simulink model "SSVEPrealtime2017"  (R2017a)
settings: Solver=VariableStepAuto  StartTime=0.0  StopTime=inf  RelTol=1e-3
libraries: dspindex x2, dspnetwork x1
settings Model: Creator=Jskyl  LastModifiedBy=a436q344
settings SFSimCC: SimUseLocalCustomCode=on
settings RTWCC: RTWUseLocalCustomCode=on

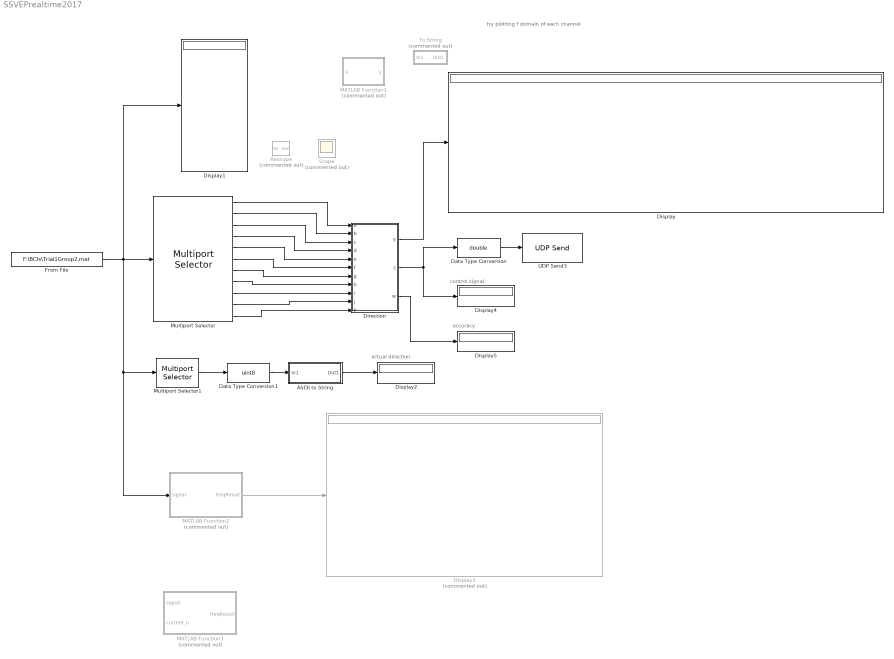
== system SSVEPrealtime2017 ==
  note: try plotting f domain of each channel
  note: actual direction
  note: accuracy
  note: control signal
  ASCII to String : Subsystem  Description=Replaced Block  mask(Replaced Block){}
      mask help: This block has been replaced with an empty subsystem because it used functionality that is unavailable in Simulink R2017a.
      mask Display: fprintf('Replaced: %s\n','ASCIIToString')
  Data Type Conversion : DataTypeConversion  OutDataTypeStr=double  ConvertRealWorld=Stored Integer (SI)
  Data Type Conversion1 : DataTypeConversion  OutDataTypeStr=uint8
  Direction : MATLAB Function  TreatAsAtomicUnit=on
  Display{,1..2,4..5} (5 alike) : Display
  Display3 : Display  Commented=on
  From File : FromFile  FileName=F:\BCIs\Trial1Group2.mat  OutDataTypeStr=double  SampleTime=1/512
  MATLAB Function1 : MATLAB Function  Commented=on  TreatAsAtomicUnit=on
  MATLAB Function2 : MATLAB Function  Commented=on  TreatAsAtomicUnit=on
  MATLAB Function3 : MATLAB Function  Commented=on  TreatAsAtomicUnit=on
  Multiport Selector : dspindex/Multiport Selector  rowsOrCols=Rows  idxCellArray={ 1,2,3,4,5,6,7,8,9,10,11 }  idxErrMode=Clip Index
  Multiport Selector1 : dspindex/Multiport Selector  rowsOrCols=Rows  idxCellArray={ 11 }  idxErrMode=Clip Index
  Reshape : Reshape  Commented=on  OutputDimensionality=Customize  OutputDimensions=[10,1]
  Scope : Scope  Commented=on
  To String : Subsystem  Description=Replaced Block  Commented=on  mask(Replaced Block){}
      mask help: This block has been replaced with an empty subsystem because it used functionality that is unavailable in Simulink R2017a.
      mask Display: fprintf('Replaced: %s\n','ToString')
  UDP Send3 : dspnetwork/UDP Send  remoteURL='127.0.0.1'  remotePort=25000  localURL='0.0.0.0'  localPortSource=Automatically determine  localPort=-1  sampletime=-1  blockPlatform=[]  separateLengthPort=0
  wires:
  Direction/1(y) -> Display/1
  From File/1 -> MATLAB Function2/1(signal), Multiport Selector1/1, Display1/1, Multiport Selector/1
  ASCII to String/1(Out1) -> Display2/1
  Multiport Selector1/1 -> Data Type Conversion1/1
  Data Type Conversion1/1 -> ASCII to String/1(In1)
  Multiport Selector/1 -> Direction/1(a)
  Multiport Selector/2 -> Direction/2(b)
  Multiport Selector/3 -> Direction/3(c)
  Multiport Selector/4 -> Direction/4(d)
  Multiport Selector/5 -> Direction/5(e)
  Multiport Selector/6 -> Direction/6(f)
  Multiport Selector/7 -> Direction/7(g)
  Multiport Selector/8 -> Direction/8(h)
  Multiport Selector/9 -> Direction/9(i)
  Multiport Selector/10 -> Direction/10(j)
  MATLAB Function2/1(freqResult) -> Display3/1
  Multiport Selector/11 -> Direction/11(k)
  Data Type Conversion/1 -> UDP Send3/1
  Direction/2(z) -> Display4/1, Data Type Conversion/1
  Direction/3(w) -> Display5/1

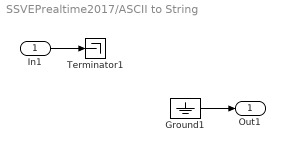
== system SSVEPrealtime2017/ASCII to String ==
  In1 : Inport
  Ground1 : Ground
  Terminator1 : Terminator
  Out1 : Outport
  wires:
  Ground1/1 -> Out1/1
  In1/1 -> Terminator1/1

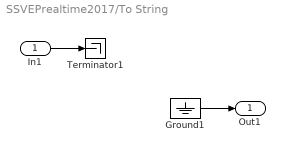
== system SSVEPrealtime2017/To String ==
  In1 : Inport
  Ground1 : Ground
  Terminator1 : Terminator
  Out1 : Outport
  wires:
  Ground1/1 -> Out1/1
  In1/1 -> Terminator1/1

== matlab function SSVEPrealtime2017/Direction ==
  data: y output size=[10 513]; a input; b input; c input; d input; e input; f input; g input; h input; i input; j input; k input; z output; w output
function [y,z,w]= fcn(a,b,c,d,e,f,g,h,i,j,k)

u = [a;b;c;d;e;f;g;h;i;j];
freq = [11 13.5 16 18.5 21 23.5 25];

persistent v
if isempty(v)
    v = 100;
end

persistent x
if isempty(x)
    x = 102;
end

persistent dir
if isempty(dir)
    dir = k;
end

persistent acc
if isempty(acc)
    acc = 0;
end

persistent keep
if isempty(keep)
   keep = 0; 
end

persistent n
if isempty(n)
    n = 0;
end

persistent mat
if isempty(mat)
    mat = u;
end

n = n + 1;
mat = [mat u]; %(1:10,n)

if k ~= 102
    dir = [dir k];
end

y = mat;

constant = 1;
sampleRate = 512;
f = constant*(0:(sampleRate/2));

%xMaxC1 = zeros(512);

if length(mat) == 513
    lowEnd = 9;
    highEnd = 31;
    filterOrder = 4; %how does this affect the outcome?
    [b,a] = butter(filterOrder, [lowEnd highEnd]/(sampleRate/2));
    data1 = filtfilt(b, a, y(1,:));
    data2 = filtfilt(b, a, y(2,:));
    data3 = filtfilt(b, a, y(3,:));
    data4 = filtfilt(b, a, y(4,:));
    data5 = filtfilt(b, a, y(5,:));
    data6 = filtfilt(b, a, y(6,:));
    data7 = filtfilt(b, a, y(7,:));
    data8 = filtfilt(b, a, y(8,:));
    data9 = filtfilt(b, a, y(9,:));
    data10 = filtfilt(b, a, y(10,:));

    y = [data1; data2; data3; data4; data5; data6; data7; data8; data9; data10];
    
    fftC1 = fft(y(1,:), 512); % C1
    pfftC1 = abs(fftC1);
    [maxC1, iMaxC1] = max(pfftC1);
    xMaxC1 = f(iMaxC1);
    fftC2 = abs(fft(y(2,:), 512)); % C2
    [maxC2, iMaxC2] = max(fftC2);
    xMaxC2 = f(iMaxC2);
    fftC3 = abs(fft(y(3,:), 512)); % C3
    [maxC3, iMaxC3] = max(fftC3);
    xMaxC3 = f(iMaxC3);
    fftC4 = abs(fft(y(4,:), 512)); % C4
    [maxC4, iMaxC4] = max(fftC4);
    xMaxC4= f(iMaxC4);
    fftC5 = abs(fft(y(5,:), 512)); % C5
    [maxC5, iMaxC5] = max(fftC5);
    xMaxC5 = f(iMaxC5);
    fftC6 = abs(fft(y(6,:), 512)); % C6
    [maxC6, iMaxC6] = max(fftC6);
    xMaxC6 = f(iMaxC6);
    fftC7 = abs(fft(y(7,:), 512)); % C7
    [maxC7, iMaxC7] = max(fftC7);
    xMaxC7 = f(iMaxC7);
    fftC8 = abs(fft(y(8,:), 512)); % C8
    [maxC8, iMaxC8] = max(fftC8);
    xMaxC8 = f(iMaxC8);
    fftC9 = abs(fft(y(9,:), 512)); % C9
    [maxC9, iMaxC9] = max(fftC9);
    xMaxC9 = f(iMaxC9);
    fftC10 = abs(fft(y(10,:), 512)); % C10
    [maxC10, iMaxC10] = max(fftC10);
    xMaxC10 = f(iMaxC10);

    xMax = [xMaxC1 xMaxC2 xMaxC3 xMaxC4 xMaxC5 xMaxC6 xMaxC7 xMaxC8 xMaxC9 xMaxC10];
    xMaxAvg = mean(xMax);
    keep = [keep xMaxAvg]
    
    %average
    
    direction = abs(xMaxAvg - freq);
    [minDirection, iDirection] = min(direction);
    
    if iDirection == 1
        z = 117;
        x = z;
        disp('up');
        if mode(dir) == 117
            acc = [acc 1];
        else
            acc = [acc 0];
        end
    end
    if iDirection == 2
        z = 105;
        x = z;
        disp('in');
        if mode(dir) == 105
            acc = [acc 1];
        else
            acc = [acc 0];
        end
    end
    if iDirection == 3
        z = 114;
        x = z;
        disp('right');
        if mode(dir) == 114
            acc = [acc 1];
        else
            acc = [acc 0];
        end
    end
    if iDirection == 4
        z = 100;
        x = z;
        disp('down');
        if mode(dir) == 100
            acc = [acc 1];
        else
            acc = [acc 0];
        end
    end
    if iDirection == 5
        z = 111;
        x = z;
        disp('out');
        if mode(dir) == 111
            acc = [acc 1];
        else
            acc = [acc 0];
        end
    end
    if iDirection == 6
        z = 108;
        x = z;
        disp('left');
        if mode(dir) == 108
            acc = [acc 1];
        else
            acc = [acc 0];
        end
    end
    if iDirection == 7
        z = 115;
        x = z;
        disp('stop');
        if mode(dir) == 115
            acc = [acc 1];
        else
            acc = [acc 0];
        end
    end
    
    %dispDir = sprintf('Direction = %f' , mode(dir));
    %disp(dispDir);
    disp(mode(dir));
    
    accuracy = 100*sum(acc)/(length(acc)-1);
    %dispAcc = sprintf('Accuracy = %.3f' , accuracy);
    %disp(accuracy);
    v = accuracy;
end

w = v;
z = x;

if n == 512
    mat = u;
    n = 0;
    dir = k;
    %acc = 0;
    %disp("done");
end

== matlab function SSVEPrealtime2017/MATLAB Function1 ==
  data: u input; y output
function y = fcn(u)

string var;

if u == 108
   var = "left";
end
if u == 102
   var = "right";
end
if u == 117
   var = "up";
end
if u == 100
   var = "down";
end
if u == 105
   var = "in";
end
if u == 111
   var = "out";
end
if u == 115
   var = "stop";
end
if u == 102
   var = "off";
end

y = double(charg(var));

== matlab function SSVEPrealtime2017/MATLAB Function2 ==
  data: signal input; freqResult output
function freqResult=MEC(signal) %current_n

signal=signal';
%% Functions Enabling 
CMA_filter=1;
FFT_HP_IFFT=1;
exp_transform=0;
mid_freqs=1;
consider_threshhold=0;

%% Defining Parameteres

f=[11 13.5 16 18.5 21 23.5 25];            %frequencies in concern
Fs = 128;           %Sampling frequency of Emotive
O1=7;               %| Name and number of channals 
O2=8;
T7=5;
T8=10;
Nh=2;               %#of Harmonics 
Ny=4;               %#of using Channals
alfa_energy_co=0.25;    %alfa as in the last section of paper#3
beta_classification=0.35;    %beta as in the last section of paper#3
valid_channal=[1 2 3 4 6 9 11 12 13 14]; %Valid Channals except using channals (O1, O2, T7 , T8) to use in CMA
cutting_freq=5;  %freq at which HP filter work

%% Calculating Needed Parameteres 
if (mid_freqs)
    %freqs in concern (including mid Freqs)
    midFreq=diff(f)/2+f(1:length(f)-1);
    f=horzcat(f,midFreq);
    %--> f=[ freqs in concern + mid freqs]
end

Nf=length(f);

%Filtering CMA
if (CMA_filter)
left_signal = double (signal (:,valid_channal));
EEG_background_signal = mean(left_signal,2);
EEG_background_signal_all= repmat(EEG_background_signal,1,Ny);
end

%Deriving subSignals and Y
yO1= double (signal (:,O1)); %for DP floating point (e.g. SVM)
yO2= double (signal (:,O2)); %Subtracting EEG background signal
yT7= double (signal (:,T7));
yT8= double (signal (:,T8));

Nt=length(yO1);

Y=zeros(Nt,Ny);
Y(:,1)=yO1;
Y(:,2)=yO2;
Y(:,3)=yT7;
Y(:,4)=yT8;  %* Here add if you want to add real channals, Also change Ny in "paramateres" 

if (CMA_filter)
    Y=Y-EEG_background_signal_all;
end

if (FFT_HP_IFFT)
    fft_Y=fft(Y);
    m_start=floor(cutting_freq/Fs*Nt+1);  
    m_end=floor(Nt-cutting_freq/Fs*Nt); 
    fft_Y(1:m_start,:)=0;
    fft_Y(m_end:Nt,:)=0;
    Y=ifft(fft_Y);
end


%% Calculating X Matris
t=linspace(0,Nt/Fs,Nt);
X=zeros(Nf,Nt,2*Nh);
for j=1:Nf
    for i=1:Nh
        X(j,:,2*i-1)=sin(2*pi*i*f(j)*t);
        X(j,:,2*i)  =cos(2*pi*i*f(j)*t);
    end
end


% Calculating Ytild
Ytild=zeros(Nf,Nt,Ny);
for i=1:Nf
    X_this_freq= squeeze(X(i,:,:));  
    Ytild(i,:,:)=Y-X_this_freq*inv(( (X_this_freq')*X_this_freq))*(X_this_freq')*Y;
end

%% Calculating Ytild_trans*Ytild=Yeig  and eigs  and W eights

Yeig=zeros(Nf,Ny,Ny);
Ns=Ny;              %#of Artificial Channals
for i=1:Nf
   Yeig(i,:,:)=(squeeze(Ytild(i,:,:)))'*squeeze(Ytild(i,:,:));
end
W=zeros(Nf,Ny,Ns);
for i=1:Nf
    [V,D]=eig(squeeze(Yeig(i,:,:)));
    eigValues=diag(D)';
    sqrt_eigValues=sqrt(eigValues);
    [sorted_eigvalues,n]=sort(sqrt_eigValues);
    sorted_vectors=V(:,n);
    W(i,:,:)=sorted_vectors./repmat(sqrt_eigValues,Ny,1) ;   
end

%% Calculating S 

S=zeros(Nf,Nt,Ns);
for i=1:Nf
   W_this=squeeze(W(i,:,:));
   S(i,:,:)=Y*W_this;
end

%% Calculating P_hat & P & P_prim

P_hat=zeros(1,Nf);
for i=1:Nf
    % for each freq
    S_this=squeeze(S(i,:,:));
    X_this=squeeze(X(i,:,:));
    for l=1:Ns
       for k=1:Nh
          P_hat(i)=P_hat(i)+ norm(X_this(:,k)'*S_this(:,l))^2;
       end
    end
    
end

P_hat=P_hat/(Ns*Nh);
%P_hat Done 

P=P_hat/sum(P_hat);
P_prim=P;
if (exp_transform)
   P_prim=exp(alfa_energy_co*P)/sum(exp(alfa_energy_co*P));    
end

name_str=sprintf('P_prim_data_%d.mat',current_n);% Just to save online datas
save(name_str,'P_prim'); 

%% Classification

[maxP_prim argmax_P_prim]=max(P_prim);
if (argmax_P_prim<=Nf)
   if (P_prim(argmax_P_prim)>=beta_classification)
      freqResult=f (argmax_P_prim);   %print out result
      return;
   else
       if (consider_threshhold==0)
            freqResult=f (argmax_P_prim);   %print out result
            return;
       end
   end
end


%% 
freqResult=0;


end

== matlab function SSVEPrealtime2017/MATLAB Function3 ==
  data: signal input; freqResult output; current_n input
function freqResult=MEC(signal,current_n)

signal=signal';
%% Functions Enabling 
CMA_filter=1;
FFT_HP_IFFT=1;
exp_transform=0;
mid_freqs=1;
consider_threshhold=0;

%% Defining Parameteres

f=[8 10 12 14 16];            %frequencies in concern
Fs = 128;           %Sampling frequency of Emotive
O1=7;               %| Name and number of channals 
O2=8;
T7=5;
T8=10;
Nh=2;               %#of Harmonics 
Ny=4;               %#of using Channals
alfa_energy_co=0.25;    %alfa as in the last section of paper#3
beta_classification=0.35;    %beta as in the last section of paper#3
valid_channal=[1 2 3 4 6 9 11 12 13 14]; %Valid Channals except using channals (O1, O2, T7 , T8) to use in CMA
cutting_freq=5;  %freq at which HP filter work

%% Calculating Needed Parameteres 
if (mid_freqs)
    %freqs in concern (including mid Freqs)
    midFreq=diff(f)/2+f(1:length(f)-1);
    f=horzcat(f,midFreq);
    %--> f=[ freqs in concern + mid freqs]
end

Nf=length(f);

%Filtering CMA
if (CMA_filter)
left_signal = double (signal (:,valid_channal));
EEG_background_signal = mean(left_signal,2);
EEG_background_signal_all= repmat(EEG_background_signal,1,Ny);
end

%Deriving subSignals and Y
yO1= double (signal (:,O1)); %for DP floating point (e.g. SVM)
yO2= double (signal (:,O2)); %Subtracting EEG background signal
yT7= double (signal (:,T7));
yT8= double (signal (:,T8));

Nt=length(yO1);

Y=zeros(Nt,Ny);
Y(:,1)=yO1;
Y(:,2)=yO2;
Y(:,3)=yT7;
Y(:,4)=yT8;  %* Here add if you want to add real channals, Also change Ny in "paramateres" 

if (CMA_filter)
    Y=Y-EEG_background_signal_all;
end

if (FFT_HP_IFFT)
    fft_Y=fft(Y);
    m_start=floor(cutting_freq/Fs*Nt+1);  
    m_end=floor(Nt-cutting_freq/Fs*Nt); 
    fft_Y(1:m_start,:)=0;
    fft_Y(m_end:Nt,:)=0;
    Y=ifft(fft_Y);
end


%% Calculating X Matris
t=linspace(0,Nt/Fs,Nt);
X=zeros(Nf,Nt,2*Nh);
for j=1:Nf
    for i=1:Nh
        X(j,:,2*i-1)=sin(2*pi*i*f(j)*t);
        X(j,:,2*i)  =cos(2*pi*i*f(j)*t);
    end
end


% Calculating Ytild
Ytild=zeros(Nf,Nt,Ny);
for i=1:Nf
    X_this_freq= squeeze(X(i,:,:));  
    Ytild(i,:,:)=Y-X_this_freq*inv(( (X_this_freq')*X_this_freq))*(X_this_freq')*Y;
end

%% Calculating Ytild_trans*Ytild=Yeig  and eigs  and W eights

Yeig=zeros(Nf,Ny,Ny);
Ns=Ny;              %#of Artificial Channals
for i=1:Nf
   Yeig(i,:,:)=(squeeze(Ytild(i,:,:)))'*squeeze(Ytild(i,:,:));
end
W=zeros(Nf,Ny,Ns);
for i=1:Nf
    [V,D]=eig(squeeze(Yeig(i,:,:)));
    eigValues=diag(D)';
    sqrt_eigValues=sqrt(eigValues);
    [sorted_eigvalues,n]=sort(sqrt_eigValues);
    sorted_vectors=V(:,n);
    W(i,:,:)=sorted_vectors./repmat(sqrt_eigValues,Ny,1) ;   
end

%% Calculating S 

S=zeros(Nf,Nt,Ns);
for i=1:Nf
   W_this=squeeze(W(i,:,:));
   S(i,:,:)=Y*W_this;
end

%% Calculating P_hat & P & P_prim

P_hat=zeros(1,Nf);
for i=1:Nf
    % for each freq
    S_this=squeeze(S(i,:,:));
    X_this=squeeze(X(i,:,:));
    for l=1:Ns
       for k=1:Nh
          P_hat(i)=P_hat(i)+ norm(X_this(:,k)'*S_this(:,l))^2;
       end
    end
    
end

P_hat=P_hat/(Ns*Nh);
%P_hat Done 

P=P_hat/sum(P_hat);
P_prim=P;
if (exp_transform)
   P_prim=exp(alfa_energy_co*P)/sum(exp(alfa_energy_co*P));    
end

name_str=sprintf('P_prim_data_%d.mat',current_n);% Just to save online datas
save(name_str,'P_prim'); 

%% Classification

[maxP_prim argmax_P_prim]=max(P_prim);
if (argmax_P_prim<=Nf)
   if (P_prim(argmax_P_prim)>=beta_classification)
      freqResult=f (argmax_P_prim);   %print out result
      return;
   else
       if (consider_threshhold==0)
            freqResult=f (argmax_P_prim);   %print out result
            return;
       end
   end
end


%% 
freqResult=0;


end
